simulink model "MRAC_generalizado"  (Simulink 10.3)
settings: Solver=ode45  StartTime=10  StopTime=20  RelTol=1e-3  AbsTol=1e-6
values from neighbouring files (symbols this model uses):
  Af = zeros(n-1,n-1)    [MRAC_generalizado.m]    (also in MRAC_generalizado_nstar_1.m = zeros(nf); Af(1:nf-1, 2:nf) = eye(nf-1); Af(end, :) = -flipl; MRAC_generalizado_nstar_2.m = zeros(nf); Af(1:nf-1, 2:nf) = eye(nf-1); Af(end, :) = -flipl)
  Aq = 2    [MRAC_generalizado_nstar_1.m]    (also in MRAC_generalizado_nstar_2.m = 5)
  As = 5    [MRAC_generalizado_nstar_1.m]    (also in MRAC_generalizado_nstar_2.m = 3)
  As2 = 2    [MRAC_generalizado_nstar_2.m]
  Bf = zeros(n-1,1)    [MRAC_generalizado.m]    (also in MRAC_generalizado_nstar_1.m = zeros(nf,1); Bf(end) = 1; MRAC_generalizado_nstar_2.m = zeros(nf,1); Bf(end) = 1)
  DC = 2    [MRAC_generalizado_nstar_1.m]    (also in MRAC_generalizado_nstar_2.m)
  gamma = 10*eye(2*n)    [MRAC_generalizado_nstar_1.m]    (also in MRAC_generalizado_nstar_2.m)
  kp = 2    [MRAC_generalizado.m]    (also in MRAC_generalizado_nstar_1.m = 2 + rand(); MRAC_generalizado_nstar_2.m; controle2DOF.m = N_p(find(N_p ~= 0, 1, 'first')); controle2DOF_nstar2.m = N_p(find(N_p ~= 0, 1, 'first')))
  st = 0.01    [MRAC_generalizado_nstar_1.m]    (also in MRAC_generalizado_nstar_2.m)
  theta0 = 0.95*theta_star    [MRAC_generalizado_nstar_1.m]    (also in MRAC_generalizado_nstar_2.m)
  wq = 0.1*pi    (= 0.314159265359)    [MRAC_generalizado_nstar_1.m]    (also in MRAC_generalizado_nstar_2.m)
  ws = 1    [MRAC_generalizado_nstar_1.m]    (also in MRAC_generalizado_nstar_2.m = 0.628318530718)
  ws2 = 0.3*pi    (= 0.942477796077)    [MRAC_generalizado_nstar_2.m]
libraries: cstblocks x2
settings Model: LogicAnalyzerSignalOrdering=91375379-6204-4e29-b584-b898db01c62f,b1c03556-8efb-47e3-8c3b-ea0d47cc8d01,995f44ca-3b1b-4533-9df6-5245141e0052  Creator=Ramon  LastModifiedBy=LRPROENC  MultithreadedSim=on
settings SolverCC: AutoScaleAbsTol=off
settings DataIOCC: SaveOutput=off  SaveTime=off
settings OptimizationCC: BlockReduction=off  BooleanDataType=off  InitFltsAndDblsToZero=on
settings DebuggingCC: SaveWithParameterizedLinksMsg=none  SignalResolutionControl=TryResolveAllWithWarning  MultiTaskDSMMsg=warning  MultiTaskCondExecSysMsg=none
settings HardwareCC: TargetUnknown=on
settings RTWCC: TemplateMakefile=grt_vc.tmf

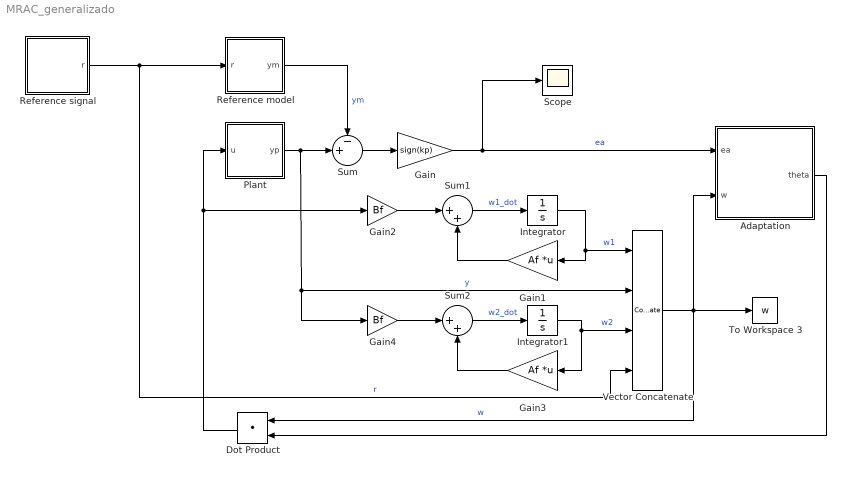
== system MRAC_generalizado ==
  Adaptation : Subsystem
  Dot Product : DotProduct  InputSameDT=on  OutDataTypeStr=Inherit: Inherit via internal rule
  Gain : Gain  Gain=sign(kp)
  Gain1 : Gain  Gain=Af  Multiplication=Matrix(K*u) (u vector)
  Gain2 : Gain  Gain=Bf
  Gain3 : Gain  Gain=Af  Multiplication=Matrix(K*u) (u vector)
  Gain4 : Gain  Gain=Bf
  Integrator : Integrator
  Integrator1 : Integrator
  Plant : Subsystem
  Reference model : Subsystem
  Reference signal : Subsystem
  Scope : Scope
  Sum : Sum  Inputs=-+|  InputSameDT=on  SaturateOnIntegerOverflow=on  OutDataTypeStr=Inherit: Same as first input
  Sum1 : Sum  Inputs=|++  InputSameDT=on  SaturateOnIntegerOverflow=on  OutDataTypeStr=Inherit: Same as first input
  Sum2 : Sum  Inputs=|++  InputSameDT=on  SaturateOnIntegerOverflow=on  OutDataTypeStr=Inherit: Same as first input
  To Workspace 3 : ToWorkspace  VariableName=w  SampleTime=st
  Vector Concatenate : Concatenate  NumInputs=4
  wires:
  Reference model/1(ym) -> Sum/1  "ym"
  Plant/1(yp) -> Gain4/1, Vector Concatenate/2, Sum/2  "y"
  Dot Product/1 -> Gain2/1, Plant/1(u)
  Adaptation/1(theta) -> Dot Product/2
  Gain/1 -> Adaptation/1(ea), Scope/1  "ea"
  Sum/1 -> Gain/1
  Sum1/1 -> Integrator/1  "w1_dot"
  Gain2/1 -> Sum1/1
  Integrator/1 -> Vector Concatenate/1, Gain1/1  "w1"
  Gain1/1 -> Sum1/2
  Sum2/1 -> Integrator1/1  "w2_dot"
  Reference signal/1(r) -> Vector Concatenate/4, Reference model/1(r)  "r"
  Integrator1/1 -> Vector Concatenate/3, Gain3/1  "w2"
  Gain3/1 -> Sum2/2
  Gain4/1 -> Sum2/1
  Vector Concatenate/1 -> Dot Product/1, To Workspace 3/1, Adaptation/2(w)  "w"

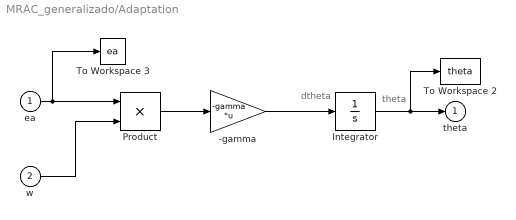
== system MRAC_generalizado/Adaptation ==
  note: theta
  note: dtheta
  ea : Inport  PortDimensions=1
  w : Inport  Port=2
  -gamma : Gain  Gain=-gamma  Multiplication=Matrix(K*u) (u vector)  SaturateOnIntegerOverflow=on  OutDataTypeStr=Inherit: Same as input  ParamDataTypeStr=Inherit: Same as input
  Integrator : Integrator  InitialCondition=theta0
  Product : Product  InputSameDT=on  RndMeth=Zero  SaturateOnIntegerOverflow=on  OutDataTypeStr=Inherit: Same as first input
  To Workspace 2 : ToWorkspace  VariableName=theta  SampleTime=st
  To Workspace 3 : ToWorkspace  VariableName=ea  SampleTime=st
  theta : Outport  InitialOutput=0  VectorParamsAs1DForOutWhenUnconnected=off
  wires:
  Integrator/1 -> To Workspace 2/1, theta/1
  -gamma/1 -> Integrator/1
  w/1 -> Product/2
  ea/1 -> Product/1, To Workspace 3/1
  Product/1 -> -gamma/1

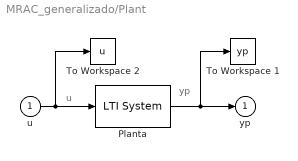
== system MRAC_generalizado/Plant ==
  note: yp
  note: u
  u : Inport
  Planta : cstblocks/LTI System  sys=P  IC=x0
  To Workspace 1 : ToWorkspace  VariableName=yp  SampleTime=st
  To Workspace 2 : ToWorkspace  VariableName=u  SampleTime=st
  yp : Outport  InitialOutput=0  VectorParamsAs1DForOutWhenUnconnected=off
  wires:
  u/1 -> To Workspace 2/1, Planta/1
  Planta/1 -> yp/1, To Workspace 1/1

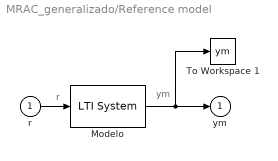
== system MRAC_generalizado/Reference model ==
  note: r
  note: ym
  r : Inport
  Modelo : cstblocks/LTI System  sys=M  IC=xm0
  To Workspace 1 : ToWorkspace  VariableName=ym  SampleTime=st
  ym : Outport  InitialOutput=0  VectorParamsAs1DForOutWhenUnconnected=off
  wires:
  Modelo/1 -> To Workspace 1/1, ym/1
  r/1 -> Modelo/1

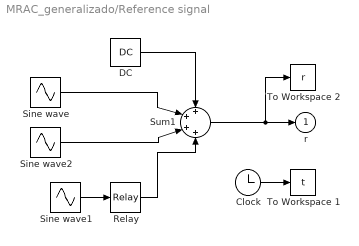
== system MRAC_generalizado/Reference signal ==
  Clock : Clock
  DC : Constant  Value=DC
  Relay : Relay  OnOutputValue=Aq  OffOutputValue=-Aq
  Sine wave : Sin  Amplitude=As  Frequency=ws  SampleTime=0
  Sine wave1 : Sin  Frequency=wq  SampleTime=0
  Sine wave2 : Sin  Amplitude=As2  Frequency=ws2  SampleTime=0
  Sum1 : Sum  Inputs=++++  InputSameDT=on  SaturateOnIntegerOverflow=on  OutDataTypeStr=Inherit: Same as first input
  To Workspace 1 : ToWorkspace  VariableName=t  SampleTime=st
  To Workspace 2 : ToWorkspace  VariableName=r  SampleTime=st
  r : Outport  InitialOutput=0  VectorParamsAs1DForOutWhenUnconnected=off
  wires:
  DC/1 -> Sum1/1
  Sum1/1 -> r/1, To Workspace 2/1
  Clock/1 -> To Workspace 1/1
  Sine wave/1 -> Sum1/2
  Relay/1 -> Sum1/4
  Sine wave1/1 -> Relay/1
  Sine wave2/1 -> Sum1/3
